simulink model "BenchmarkModel_Phasor_TestCase"  (R2020a)
settings: Solver=daessc  StartTime=0.0  StopTime=24*3600  RelTol=1e-2
undefined symbols (not defined in the file): A, a, Ac, B, Bc, C, Cc, Dc, Dd, find_system, Fnom, gcbh, I21_init_imag, I21_init_real, Ibase1, Ibase2, Iw1A_init_mag, Iw1A_init_pha, Iw1B_init_mag, Iw1B_init_pha, Iw1C_init_mag, Iw1C_init_pha, Iw2A_init_mag, Iw2A_init_pha, Iw2B_init_mag, Iw2B_init_pha, Iw2C_init_mag, Iw2C_init_pha, j, kr, ks, Nmax, Pnom, psi, sps_rtmsupport, V2G, Vnom1, Vnom2, w, Z1pu, Z2pu, Ztpu
libraries: powerlib x66, simulink x7, powerlib_meascontrol x7
(part 1 of 3)
settings Model: Creator=user  LastModifiedBy=anton
settings SolverCC: ZeroCrossControl=DisableAll

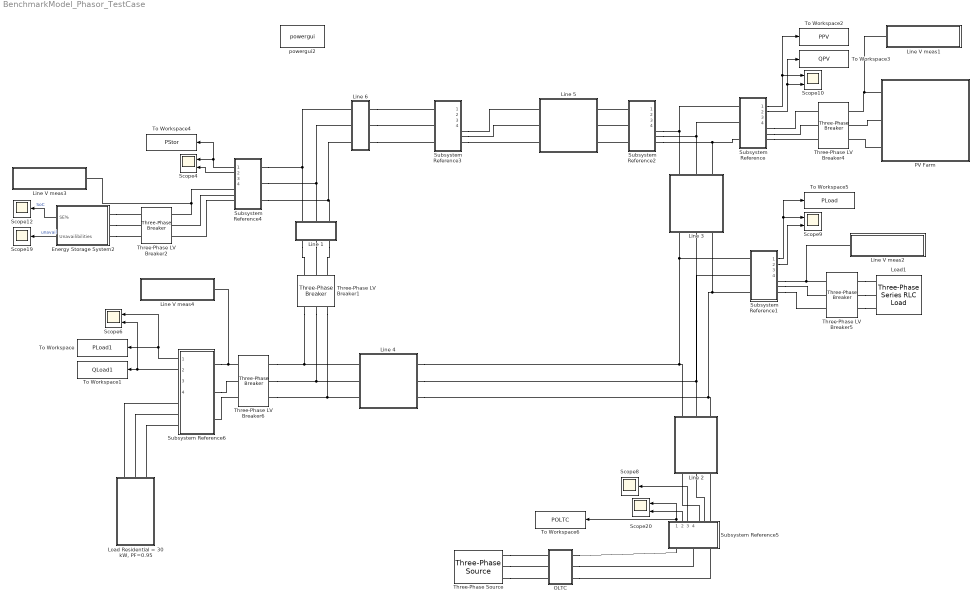
== system BenchmarkModel_Phasor_TestCase ==
  Energy Storage System2 : Subsystem  mask(Generic Energy Storage System){Pnom=15, kWh_Rated=75, Initial_kWh_pc=50, Efficiency=96, Pmax_Grid=27.5, Ki=100, MinMax=[ 10  90 ], ChargingPower=27.5}
      mask prompts: Pnom "Rated power in kW"; kWh_Rated "Rated capacity in kWh"; Initial_kWh_pc "Initial stored energy in % of rated capacity"; Efficiency "System efficiency in %"; Pmax_Grid "Maximum power allowed from the grid (kW)"; Ki "Regulator integral gain:"; MinMax "Range of operation [ min  max ] in % of Stored Energy"; ChargingPower "Maximum charging power (kW) during night time:"
      mask help:
      | Model a generic Energy Storage System (ESS) connected to grid through an inverter. The storage technology can be Battery, Flywheel, SuperCapacitor, ...
      |
      | Look Under Mask to see how the model is built.
      mask init:
      | Min=MinMax(1);
      | Max=MinMax(2);
      | Plimit=Pnom*1e3;
      mask DialogControl Container4 Prompt: Power
      mask DialogControl Container7 Prompt: Control
      mask Display: image(imread('Energy.jpg'))
  Line 1 : Subsystem  mask{Rline=0.497*3, Lline=0.086*3/(2*pi*50)}
      mask prompts: Rline "Resistance"; Lline "Reactance"
      mask DialogControl DescTextVar Prompt: Line block for LV grid
  Line 2 : Subsystem  mask{Rline=0.497*0.5, Lline=0.086*0.5/(2*pi*50)}
      mask prompts: Rline "Resistance"; Lline "Reactance"
      mask DialogControl DescTextVar Prompt: Line block for LV grid
  Line 3 : Subsystem  mask{Rline=0.497*2, Lline=0.086*2/(2*pi*50)}
      mask prompts: Rline "Resistance"; Lline "Reactance"
      mask DialogControl DescTextVar Prompt: Line block for LV grid
  Line 4 : Subsystem  mask{Rline=0.497*3, Lline=0.086*3/(2*pi*50)}
      mask prompts: Rline "Resistance"; Lline "Reactance"
      mask DialogControl DescTextVar Prompt: Line block for LV grid
  Line 5 : Subsystem  mask{Rline=0.497, Lline=0.086/(2*pi*50)}
      mask prompts: Rline "Resistance"; Lline "Reactance"
      mask DialogControl DescTextVar Prompt: Line block for LV grid
  Line 6 : Subsystem  mask{Rline=0.497, Lline=0.086/(2*pi*50)}
      mask prompts: Rline "Resistance"; Lline "Reactance"
      mask DialogControl DescTextVar Prompt: Line block for LV grid
  Line V meas1 : Subsystem
  Line V meas2 : Subsystem
  Line V meas3 : Subsystem
  Line V meas4 : Subsystem
  "Load Residential = 30 kW, PF=0.95" : Subsystem
      mask Display: image(imread('load.jpg'))
  Load1 : powerlib/Elements/Three-Phase Series RLC Load  LConnTagsString=A|B|C  Configuration=Y (grounded)  NominalVoltage=420  Vabc=[1e3 1e3 1e3]  Vabcp=[1e3 1e3 1e3]  NominalFrequency=50  UnbalancedPower=off  ActivePower=10e3  InductivePower=1e3  CapacitivePower=0  Pabc=[10e3 9e3 11e3]  QLabc=[100 90 110]  QCabc=[100 90 110]  Pabcp=[10e3 9e3 11e3]  QLabcp=[100 90 110]  QCabcp=[100 90 110]  Measurements=None  LoadType=constant Z
  OLTC : Subsystem
  PV Farm : Subsystem
      mask Display: image(imread('PV_Farm.jpg'))
  Scope{4,6,9..10,20} (5 alike) : Scope  NumInputPorts=2
  Scope12 : Scope
  Scope19 : Scope
  Scope8 : Scope
  Subsystem Reference{,1..6} (7 alike) : Subsystem  ReferencedSubsystem=Bus_phasor
  Three-Phase LV Breaker1 : powerlib/Elements/Three-Phase Breaker  InitialState=closed  SwitchA=on  SwitchB=on  SwitchC=on  SwitchTimes=[10*3600 10*3600+880]  External=off  BreakerResistance=0.001  SnubberResistance=1e5  SnubberCapacitance=inf  Measurements=None
  Three-Phase LV Breaker2 : powerlib/Elements/Three-Phase Breaker  InitialState=closed  SwitchA=on  SwitchB=on  SwitchC=on  SwitchTimes=1e9  External=off  BreakerResistance=0.001  SnubberResistance=1e5  SnubberCapacitance=inf  Measurements=None
  Three-Phase LV Breaker4 : powerlib/Elements/Three-Phase Breaker  InitialState=closed  SwitchA=on  SwitchB=on  SwitchC=on  SwitchTimes=25*3600  External=off  BreakerResistance=0.001  SnubberResistance=1e5  SnubberCapacitance=inf  Measurements=None
  Three-Phase LV Breaker5 : powerlib/Elements/Three-Phase Breaker  InitialState=closed  SwitchA=on  SwitchB=on  SwitchC=on  SwitchTimes=20*3600  External=off  BreakerResistance=0.001  SnubberResistance=1e5  SnubberCapacitance=inf  Measurements=None
  Three-Phase LV Breaker6 : powerlib/Elements/Three-Phase Breaker  InitialState=closed  SwitchA=on  SwitchB=on  SwitchC=on  SwitchTimes=1e10  External=off  BreakerResistance=0.001  SnubberResistance=1e5  SnubberCapacitance=inf  Measurements=None
  Three-Phase Source : powerlib/Electrical Sources/Three-Phase Source  InternalConnection=Yg  VoltagePhases=off  Voltage=20e3  PhaseAngle=0  Voltage_phases=[25e3 25e3 25e3]/sqrt(3)  PhaseAngles_phases=[0 -120 +120]  Frequency=50  NonIdealSource=on  SpecifyImpedance=off  Resistance=0.6145770  Inductance=0.00163022  ShortCircuitLevel=100e6  BaseVoltage=20e3  XRratio=7  BusType=swing  Pref=10e3  Qref=0  Prefabc=[10e3, 10e3, 10e3]  Qrefabc=[0, 0, 0]  Qmin=-inf  Qmax=inf
  To Workspace : ToWorkspace  VariableName=PLoad1  SaveFormat=Timeseries  SampleTime=-1
  To Workspace1 : ToWorkspace  VariableName=QLoad1  SaveFormat=Timeseries  SampleTime=-1
  To Workspace2 : ToWorkspace  VariableName=PPV  SaveFormat=Timeseries  SampleTime=-1
  To Workspace3 : ToWorkspace  VariableName=QPV  SaveFormat=Timeseries  SampleTime=-1
  To Workspace4 : ToWorkspace  VariableName=PStor  SaveFormat=Timeseries  SampleTime=-1
  To Workspace5 : ToWorkspace  VariableName=PLoad  SaveFormat=Timeseries  SampleTime=-1
  To Workspace6 : ToWorkspace  VariableName=POLTC  SaveFormat=Timeseries  SampleTime=-1
  powergui2 : powerlib/powergui  Priority=1  SimulationMode=Phasor  SampleTime=50e-6  frequency=50  Iterations=50  frequencyindice=50  Pbase=100e6  ErrMax=1e-4  UnitsV=kV  UnitsW=MW  buscounter=0  FunctionMessages=off  echomessages=off  EnableUseOfTLC=off  CurrentSourceSwitches=off  DisableSnubberDevices=off  DisableRonSwitches=off  DisableVfSwitches=off  DisplayEquations=off  AutomaticDiscreteSolvers=off  SolverType=Tustin/Backward Euler (TBE)  Interpol=off  ExternalGateDelay=off  methode=off  Ts=100  x0status=blocks  SPID=on  SwTol=0  HookPort=off  NonlinearTolerance=1e-4  nMaxIteration=100  ContinueOnMaxIteration=off  RestoreLinks=warning  ResistiveCurrentMeasurement=off  Frange=[0:2:500]  Ylog=off  Xlog=on  ShowGrid=off  save=off  variable=ZData  structure=0  ZoomFFT=off  StartTime=0.0  cycles=1  DisplayStyle=1  fundamental=60  FreqAxis=off  MaxFrequency=1000  frequencyindicesteady=1  RmsSteady=1  display=off
  wires:
  Subsystem Reference4/1 -> To Workspace4/1, Scope4/1
  Subsystem Reference4/2 -> Scope4/2
  Subsystem Reference1/2 -> Scope9/2
  Subsystem Reference1/1 -> To Workspace5/1, Scope9/1
  Subsystem Reference/1 -> To Workspace2/1, Scope10/1
  Subsystem Reference/2 -> To Workspace3/1, Scope10/2
  Energy Storage System2/1(SE%) -> Scope12/1  "SoC"
  Energy Storage System2/2(Unavailibilities) -> Scope19/1  "unavail"
  Subsystem Reference5/1 -> Scope20/1, To Workspace6/1
  Subsystem Reference5/2 -> Scope20/2
  Subsystem Reference6/1 -> Scope6/1, To Workspace/1
  Subsystem Reference6/2 -> Scope6/2, To Workspace1/1
  Subsystem Reference5/3 -> Scope8/1
  connections:
  Subsystem Reference2/RConn2 -- Subsystem Reference/LConn2 -- Line 3/LConn2
  Subsystem Reference1/LConn3 -- Line 4/LConn3 -- Line 2/LConn3 -- Line 3/RConn3
  OLTC/RConn2 -- Subsystem Reference5/LConn2
  OLTC/RConn3 -- Subsystem Reference5/LConn3
  Subsystem Reference3/RConn3 -- Line 5/RConn3
  Subsystem Reference3/RConn2 -- Line 5/RConn2
  Subsystem Reference3/RConn1 -- Line 5/RConn1
  Subsystem Reference2/LConn3 -- Line 5/LConn3
  Subsystem Reference2/LConn2 -- Line 5/LConn2
  Subsystem Reference2/LConn1 -- Line 5/LConn1
  Subsystem Reference4/LConn3 -- Line 6/LConn3 -- Line 1/LConn3
  Subsystem Reference4/LConn2 -- Line 1/LConn2 -- Line 6/LConn2
  Subsystem Reference4/LConn1 -- Line 1/LConn1 -- Line 6/LConn1
  Line 1/RConn2 -- Three-Phase LV Breaker1/RConn2
  Line 1/RConn1 -- Three-Phase LV Breaker1/RConn1
  Line 1/RConn3 -- Three-Phase LV Breaker1/RConn3
  Subsystem Reference2/RConn1 -- Subsystem Reference/LConn1 -- Line 3/LConn1
  Three-Phase LV Breaker1/LConn2 -- Three-Phase LV Breaker6/RConn2 -- Line 4/RConn2
  Three-Phase LV Breaker1/LConn1 -- Line 4/RConn1 -- Three-Phase LV Breaker6/RConn1
  Three-Phase LV Breaker1/LConn3 -- Line 4/RConn3 -- Three-Phase LV Breaker6/RConn3
  Energy Storage System2/LConn1 -- Three-Phase LV Breaker2/LConn1
  Energy Storage System2/LConn2 -- Three-Phase LV Breaker2/LConn2
  Energy Storage System2/LConn3 -- Three-Phase LV Breaker2/LConn3
  Subsystem Reference4/RConn1 -- Line V meas3/LConn1 -- Three-Phase LV Breaker2/RConn1
  Subsystem Reference4/RConn2 -- Three-Phase LV Breaker2/RConn2
  Subsystem Reference4/RConn3 -- Three-Phase LV Breaker2/RConn3
  PV Farm/RConn2 -- Three-Phase LV Breaker4/LConn2
  PV Farm/RConn3 -- Three-Phase LV Breaker4/LConn3
  Subsystem Reference/RConn1 -- Three-Phase LV Breaker4/RConn1
  Subsystem Reference/RConn2 -- Three-Phase LV Breaker4/RConn2
  Subsystem Reference/RConn3 -- Three-Phase LV Breaker4/RConn3
  Three-Phase LV Breaker5/LConn1 -- Load1/LConn1
  Three-Phase LV Breaker5/LConn2 -- Load1/LConn2
  Three-Phase LV Breaker5/LConn3 -- Load1/LConn3
  Subsystem Reference1/RConn1 -- Line V meas2/LConn1 -- Three-Phase LV Breaker5/RConn1
  Subsystem Reference1/RConn2 -- Three-Phase LV Breaker5/RConn2
  Subsystem Reference1/RConn3 -- Three-Phase LV Breaker5/RConn3
  "Load Residential = 30 kW, PF=0.95"/LConn1 -- Subsystem Reference6/RConn1
  "Load Residential = 30 kW, PF=0.95"/LConn2 -- Subsystem Reference6/RConn2
  "Load Residential = 30 kW, PF=0.95"/LConn3 -- Subsystem Reference6/RConn3
  Three-Phase Source/RConn1 -- OLTC/LConn1
  Three-Phase Source/RConn2 -- OLTC/LConn2
  Three-Phase Source/RConn3 -- OLTC/LConn3
  Subsystem Reference6/LConn1 -- Line V meas4/LConn1 -- Three-Phase LV Breaker6/LConn1
  Subsystem Reference6/LConn2 -- Three-Phase LV Breaker6/LConn2
  Subsystem Reference6/LConn3 -- Three-Phase LV Breaker6/LConn3
  PV Farm/RConn1 -- Line V meas1/LConn1 -- Three-Phase LV Breaker4/LConn1
  Subsystem Reference5/RConn3 -- Line 2/RConn3
  Subsystem Reference5/RConn2 -- Line 2/RConn2
  Subsystem Reference5/RConn1 -- Line 2/RConn1
  Line 2/LConn1 -- Subsystem Reference1/LConn1 -- Line 3/RConn1 -- Line 4/LConn1
  Subsystem Reference2/RConn3 -- Line 3/LConn3 -- Subsystem Reference/LConn3
  Line 4/LConn2 -- Subsystem Reference1/LConn2 -- Line 3/RConn2 -- Line 2/LConn2
  Line 6/RConn1 -- Subsystem Reference3/LConn1
  Line 6/RConn2 -- Subsystem Reference3/LConn2
  Line 6/RConn3 -- Subsystem Reference3/LConn3
  OLTC/RConn1 -- Subsystem Reference5/LConn1

== system BenchmarkModel_Phasor_TestCase/Energy Storage System2 ==
  Compute number of unavailibilities : Subsystem
  ESS Control : Subsystem
  Gain : Gain  Gain=-1
  Inverter (Phasor) : Subsystem
  On=1 : Step  Time=0.01*24*60*60  Before=1  SampleTime=0
  Saturation : Saturate  UpperLimit=Pnom*1e3  LowerLimit=-Pnom*1e3
  Scope : Scope
  Stored Energy Calculation (%) : Subsystem
  A : PMIOPort  Tag=PMCPort  Side=Left
  B : PMIOPort  Tag=PMCPort  Port=2  Side=Left
  C : PMIOPort  Tag=PMCPort  Port=3  Side=Left
  SE% : Outport
  Unavailibilities : Outport  Port=2
  wires:
  Saturation/1 -> Gain/1, Inverter (Phasor)/1(Power), Stored Energy Calculation (%)/1(Pin), Compute number of unavailibilities/2(Sat Out)
  ESS Control/1(P) -> Saturation/1, Compute number of unavailibilities/1(Sat In)
  [Vabc_B1] -> ESS Control/1(Vabc)
  [Iabc_B1] -> ESS Control/2(Iabc)
  On=1/1 -> ESS Control/3(On)
  ESS Control/2(LessThan Min) -> Compute number of unavailibilities/3(LessThanMin)
  Compute number of unavailibilities/1(Unavailibilities) -> Unavailibilities/1
  Stored Energy Calculation (%)/1(SE%) -> SE%/1, ESS Control/4(SE%)
  Gain/1 -> Scope/1
  connections:
  Inverter (Phasor)/RConn1 -- A/RConn1
  Inverter (Phasor)/RConn2 -- B/RConn1
  Inverter (Phasor)/RConn3 -- C/RConn1

== system BenchmarkModel_Phasor_TestCase/Line 1 ==
  Series RLC BranchA : powerlib/Elements/Series RLC Branch  LConnTagsString=__new0  RConnTagsString=__new0  BranchType=RL  Resistance=Rline  Inductance=Lline  SetiL0=off  InitialCurrent=0  Capacitance=1e-6  Setx0=off  InitialVoltage=0  Measurements=None
  Series RLC BranchB : powerlib/Elements/Series RLC Branch  LConnTagsString=__new0  RConnTagsString=__new0  BranchType=RL  Resistance=Rline  Inductance=Lline  SetiL0=off  InitialCurrent=0  Capacitance=1e-6  Setx0=off  InitialVoltage=0  Measurements=None
  Series RLC BranchC : powerlib/Elements/Series RLC Branch  LConnTagsString=__new0  RConnTagsString=__new0  BranchType=RL  Resistance=Rline  Inductance=Lline  SetiL0=off  InitialCurrent=0  Capacitance=1e-6  Setx0=off  InitialVoltage=0  Measurements=None
  a : PMIOPort  Side=Left
  A : PMIOPort  Port=2  Side=Right
  b : PMIOPort  Port=3  Side=Left
  B : PMIOPort  Port=4  Side=Right
  c : PMIOPort  Port=5  Side=Left
  C : PMIOPort  Port=6  Side=Right
  connections:
  Series RLC BranchB/RConn1 -- B/RConn1
  Series RLC BranchC/RConn1 -- C/RConn1
  Series RLC BranchB/LConn1 -- b/RConn1
  Series RLC BranchA/RConn1 -- A/RConn1
  Series RLC BranchA/LConn1 -- a/RConn1
  Series RLC BranchC/LConn1 -- c/RConn1

== system BenchmarkModel_Phasor_TestCase/Line 2 ==
  Series RLC BranchA : powerlib/Elements/Series RLC Branch  LConnTagsString=__new0  RConnTagsString=__new0  BranchType=RL  Resistance=Rline  Inductance=Lline  SetiL0=off  InitialCurrent=0  Capacitance=1e-6  Setx0=off  InitialVoltage=0  Measurements=None
  Series RLC BranchB : powerlib/Elements/Series RLC Branch  LConnTagsString=__new0  RConnTagsString=__new0  BranchType=RL  Resistance=Rline  Inductance=Lline  SetiL0=off  InitialCurrent=0  Capacitance=1e-6  Setx0=off  InitialVoltage=0  Measurements=None
  Series RLC BranchC : powerlib/Elements/Series RLC Branch  LConnTagsString=__new0  RConnTagsString=__new0  BranchType=RL  Resistance=Rline  Inductance=Lline  SetiL0=off  InitialCurrent=0  Capacitance=1e-6  Setx0=off  InitialVoltage=0  Measurements=None
  a : PMIOPort  Side=Left
  A : PMIOPort  Port=2  Side=Right
  b : PMIOPort  Port=3  Side=Left
  B : PMIOPort  Port=4  Side=Right
  c : PMIOPort  Port=5  Side=Left
  C : PMIOPort  Port=6  Side=Right
  connections:
  Series RLC BranchC/LConn1 -- c/RConn1
  Series RLC BranchA/LConn1 -- a/RConn1
  Series RLC BranchA/RConn1 -- A/RConn1
  Series RLC BranchB/LConn1 -- b/RConn1
  Series RLC BranchC/RConn1 -- C/RConn1
  Series RLC BranchB/RConn1 -- B/RConn1

== system BenchmarkModel_Phasor_TestCase/Line 3 ==
  Series RLC BranchA : powerlib/Elements/Series RLC Branch  LConnTagsString=__new0  RConnTagsString=__new0  BranchType=RL  Resistance=Rline  Inductance=Lline  SetiL0=off  InitialCurrent=0  Capacitance=1e-6  Setx0=off  InitialVoltage=0  Measurements=None
  Series RLC BranchB : powerlib/Elements/Series RLC Branch  LConnTagsString=__new0  RConnTagsString=__new0  BranchType=RL  Resistance=Rline  Inductance=Lline  SetiL0=off  InitialCurrent=0  Capacitance=1e-6  Setx0=off  InitialVoltage=0  Measurements=None
  Series RLC BranchC : powerlib/Elements/Series RLC Branch  LConnTagsString=__new0  RConnTagsString=__new0  BranchType=RL  Resistance=Rline  Inductance=Lline  SetiL0=off  InitialCurrent=0  Capacitance=1e-6  Setx0=off  InitialVoltage=0  Measurements=None
  a : PMIOPort  Side=Left
  A : PMIOPort  Port=2  Side=Right
  b : PMIOPort  Port=3  Side=Left
  B : PMIOPort  Port=4  Side=Right
  c : PMIOPort  Port=5  Side=Left
  C : PMIOPort  Port=6  Side=Right
  connections:
  Series RLC BranchB/RConn1 -- B/RConn1
  Series RLC BranchC/RConn1 -- C/RConn1
  Series RLC BranchB/LConn1 -- b/RConn1
  Series RLC BranchA/RConn1 -- A/RConn1
  Series RLC BranchA/LConn1 -- a/RConn1
  Series RLC BranchC/LConn1 -- c/RConn1

== system BenchmarkModel_Phasor_TestCase/Line 4 ==
  Series RLC BranchA : powerlib/Elements/Series RLC Branch  LConnTagsString=__new0  RConnTagsString=__new0  BranchType=RL  Resistance=Rline  Inductance=Lline  SetiL0=off  InitialCurrent=0  Capacitance=1e-6  Setx0=off  InitialVoltage=0  Measurements=None
  Series RLC BranchB : powerlib/Elements/Series RLC Branch  LConnTagsString=__new0  RConnTagsString=__new0  BranchType=RL  Resistance=Rline  Inductance=Lline  SetiL0=off  InitialCurrent=0  Capacitance=1e-6  Setx0=off  InitialVoltage=0  Measurements=None
  Series RLC BranchC : powerlib/Elements/Series RLC Branch  LConnTagsString=__new0  RConnTagsString=__new0  BranchType=RL  Resistance=Rline  Inductance=Lline  SetiL0=off  InitialCurrent=0  Capacitance=1e-6  Setx0=off  InitialVoltage=0  Measurements=None
  a : PMIOPort  Side=Left
  A : PMIOPort  Port=2  Side=Right
  b : PMIOPort  Port=3  Side=Left
  B : PMIOPort  Port=4  Side=Right
  c : PMIOPort  Port=5  Side=Left
  C : PMIOPort  Port=6  Side=Right
  connections:
  Series RLC BranchB/RConn1 -- B/RConn1
  Series RLC BranchC/RConn1 -- C/RConn1
  Series RLC BranchB/LConn1 -- b/RConn1
  Series RLC BranchA/RConn1 -- A/RConn1
  Series RLC BranchA/LConn1 -- a/RConn1
  Series RLC BranchC/LConn1 -- c/RConn1

== system BenchmarkModel_Phasor_TestCase/Line 5 ==
  Series RLC BranchA : powerlib/Elements/Series RLC Branch  LConnTagsString=__new0  RConnTagsString=__new0  BranchType=RL  Resistance=Rline  Inductance=Lline  SetiL0=off  InitialCurrent=0  Capacitance=1e-6  Setx0=off  InitialVoltage=0  Measurements=None
  Series RLC BranchB : powerlib/Elements/Series RLC Branch  LConnTagsString=__new0  RConnTagsString=__new0  BranchType=RL  Resistance=Rline  Inductance=Lline  SetiL0=off  InitialCurrent=0  Capacitance=1e-6  Setx0=off  InitialVoltage=0  Measurements=None
  Series RLC BranchC : powerlib/Elements/Series RLC Branch  LConnTagsString=__new0  RConnTagsString=__new0  BranchType=RL  Resistance=Rline  Inductance=Lline  SetiL0=off  InitialCurrent=0  Capacitance=1e-6  Setx0=off  InitialVoltage=0  Measurements=None
  a : PMIOPort  Side=Left
  A : PMIOPort  Port=2  Side=Right
  b : PMIOPort  Port=3  Side=Left
  B : PMIOPort  Port=4  Side=Right
  c : PMIOPort  Port=5  Side=Left
  C : PMIOPort  Port=6  Side=Right
  connections:
  Series RLC BranchB/RConn1 -- B/RConn1
  Series RLC BranchC/RConn1 -- C/RConn1
  Series RLC BranchB/LConn1 -- b/RConn1
  Series RLC BranchA/RConn1 -- A/RConn1
  Series RLC BranchA/LConn1 -- a/RConn1
  Series RLC BranchC/LConn1 -- c/RConn1

== system BenchmarkModel_Phasor_TestCase/Line 6 ==
  Series RLC BranchA : powerlib/Elements/Series RLC Branch  LConnTagsString=__new0  RConnTagsString=__new0  BranchType=RL  Resistance=Rline  Inductance=Lline  SetiL0=off  InitialCurrent=0  Capacitance=1e-6  Setx0=off  InitialVoltage=0  Measurements=None
  Series RLC BranchB : powerlib/Elements/Series RLC Branch  LConnTagsString=__new0  RConnTagsString=__new0  BranchType=RL  Resistance=Rline  Inductance=Lline  SetiL0=off  InitialCurrent=0  Capacitance=1e-6  Setx0=off  InitialVoltage=0  Measurements=None
  Series RLC BranchC : powerlib/Elements/Series RLC Branch  LConnTagsString=__new0  RConnTagsString=__new0  BranchType=RL  Resistance=Rline  Inductance=Lline  SetiL0=off  InitialCurrent=0  Capacitance=1e-6  Setx0=off  InitialVoltage=0  Measurements=None
  a : PMIOPort  Side=Left
  A : PMIOPort  Port=2  Side=Right
  b : PMIOPort  Port=3  Side=Left
  B : PMIOPort  Port=4  Side=Right
  c : PMIOPort  Port=5  Side=Left
  C : PMIOPort  Port=6  Side=Right
  connections:
  Series RLC BranchB/RConn1 -- B/RConn1
  Series RLC BranchC/RConn1 -- C/RConn1
  Series RLC BranchB/LConn1 -- b/RConn1
  Series RLC BranchA/RConn1 -- A/RConn1
  Series RLC BranchA/LConn1 -- a/RConn1
  Series RLC BranchC/LConn1 -- c/RConn1

== system BenchmarkModel_Phasor_TestCase/Line V meas1 ==
  To Workspace4 : ToWorkspace  VariableName=VmagPV  SaveFormat=Timeseries  SampleTime=-1
  Va (V)2 : Scope
  Va2 : powerlib/Measurements/Voltage Measurement  Tag=PoWeRsYsTeMmEaSuReMeNt  PhasorSimulation=on  OutputType=Magnitude  PSBequivalent=0
  output Ground3 : powerlib/Elements/Ground  LConnTagsString=a
  + : PMIOPort  Side=Left
  wires:
  Va2/1 -> To Workspace4/1, Va (V)2/1  "ASM terminal voltage"
  connections:
  output Ground3/LConn1 -- Va2/LConn2
  Va2/LConn1 -- +/RConn1

== system BenchmarkModel_Phasor_TestCase/Line V meas2 ==
  To Workspace4 : ToWorkspace  VariableName=VmagLoad  SaveFormat=Timeseries  SampleTime=-1
  Va (V)2 : Scope
  Va2 : powerlib/Measurements/Voltage Measurement  Tag=PoWeRsYsTeMmEaSuReMeNt  PhasorSimulation=on  OutputType=Magnitude  PSBequivalent=0
  output Ground3 : powerlib/Elements/Ground  LConnTagsString=a
  + : PMIOPort  Side=Left
  wires:
  Va2/1 -> To Workspace4/1, Va (V)2/1  "ASM terminal voltage"
  connections:
  output Ground3/LConn1 -- Va2/LConn2
  Va2/LConn1 -- +/RConn1

== system BenchmarkModel_Phasor_TestCase/Line V meas3 ==
  To Workspace4 : ToWorkspace  VariableName=VmagStor  SaveFormat=Timeseries  SampleTime=-1
  Va (V)2 : Scope
  Va2 : powerlib/Measurements/Voltage Measurement  Tag=PoWeRsYsTeMmEaSuReMeNt  PhasorSimulation=on  OutputType=Magnitude  PSBequivalent=0
  output Ground3 : powerlib/Elements/Ground  LConnTagsString=a
  + : PMIOPort  Side=Left
  wires:
  Va2/1 -> To Workspace4/1, Va (V)2/1  "ASM terminal voltage"
  connections:
  output Ground3/LConn1 -- Va2/LConn2
  Va2/LConn1 -- +/RConn1

== system BenchmarkModel_Phasor_TestCase/Line V meas4 ==
  To Workspace4 : ToWorkspace  VariableName=VmagLoad1  SaveFormat=Timeseries  SampleTime=-1
  Va (V)2 : Scope
  Va2 : powerlib/Measurements/Voltage Measurement  Tag=PoWeRsYsTeMmEaSuReMeNt  PhasorSimulation=on  OutputType=Magnitude  PSBequivalent=0
  output Ground3 : powerlib/Elements/Ground  LConnTagsString=a
  + : PMIOPort  Side=Left
  wires:
  Va2/1 -> To Workspace4/1, Va (V)2/1  "ASM terminal voltage"
  connections:
  output Ground3/LConn1 -- Va2/LConn2
  Va2/LConn1 -- +/RConn1

== system BenchmarkModel_Phasor_TestCase/Load Residential = 30 kW, PF=0.95 ==
  Residential Load1 : Subsystem  mask{nomPower=30, PF=0.95, timestep=15}
      mask prompts: nomPower "Nominal Power (kW)"; PF "Power factor"; timestep "Timestep (minutes)"
      mask DialogControl DescGroupVar Prompt: Load profile
      mask DialogControl DescTextVar Prompt: The load profile allows you to fix a nominal power and and a power factor. It is also needed to specify the timestep used for the consumption datas. Finally, a vector expresses the consumption profile. It has to be expressed in per unit. It is imperative that the length of the vector fits with the timestep used.
      mask Display: image(imread('Residential.jpg'))
  A : PMIOPort  Side=Left
  B : PMIOPort  Port=2  Side=Left
  C : PMIOPort  Port=3  Side=Left
  connections:
  Residential Load1/LConn1 -- A/RConn1
  Residential Load1/LConn2 -- B/RConn1
  Residential Load1/LConn3 -- C/RConn1

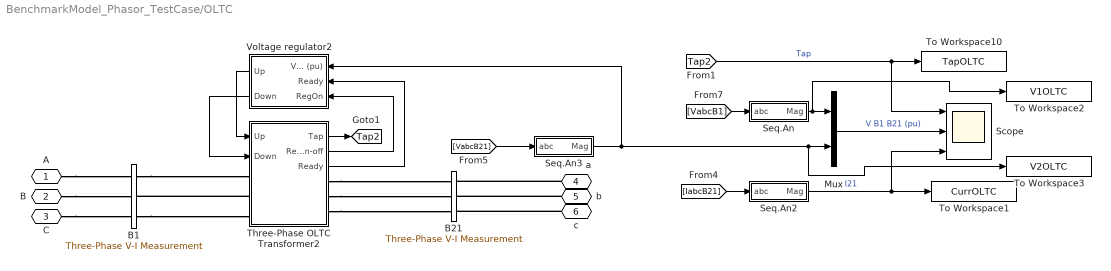
== system BenchmarkModel_Phasor_TestCase/OLTC ==
  B1 : powerlib/Measurements/Three-Phase V-I Measurement  VoltageMeasurement=phase-to-ground  SetLabelV=on  LabelV=VabcB1  Vpu=on  VpuLL=off  CurrentMeasurement=yes  SetLabelI=on  LabelI=IabcB1  Ipu=on  Pbase=630e3  Vbase=20000  OutputType=Complex  PhasorSimulation=on  PSBequivalent=0
  B21 : powerlib/Measurements/Three-Phase V-I Measurement  VoltageMeasurement=phase-to-ground  SetLabelV=on  LabelV=VabcB21  Vpu=on  VpuLL=off  CurrentMeasurement=yes  SetLabelI=on  LabelI=IabcB21  Ipu=on  Pbase=630e3  Vbase=420  OutputType=Complex  PhasorSimulation=on  PSBequivalent=0
  Mux : Mux  Inputs=2
  Scope : Scope  NumInputPorts=3
  Seq.An : Subsystem
  Seq.An2 : Subsystem
  Seq.An3 : Subsystem
  Three-Phase OLTC Transformer2 : Subsystem  AncestorBlock=|  DialogController=POWERSYS.PowerSysDialog  LoadFcn=sps_rtmsupport('LoadFcn',gcbh); %find_system(gcs,'FollowLinks', 'on', 'LookUnderMasks', 'all');  StartFcn=sps_rtmsupport('StartFcn',gcbh);  StopFcn=sps_rtmsupport('StopFcn',gcbh);  mask(Three-Phase OLTC Regulating Transformer (Phasor Type)){Winding1Connection=Delta (D11), Winding2Connection=Y, PnomFnom=[250e3  50], Winding1=[20000  0.003 0.09 ], Winding2=[420   0.003 0.09 ], Iw2_init=[0.15 -50], RmXm=[300 300], TapOnWinding=Winding 1, WindingTap=[ 0.003 0.09], dU=0.01875/5, TapMinMax=[ -8  +8], InitialTap=-4, TapSelectionTime=10, ExternalControl=on, RegulatorOn=on, Regulator=[1.04   0.0375 1]}
      | spsThreePhaseOLTCRegulatingTransformerPhasorTypeLib/Three-Phase OLTC
      | Regulating Transformer
      | (Phasor Type)
      mask prompts: Winding1Connection "Winding 1 connection (ABC terminals):"; Winding2Connection "Winding 2 connection (abc terminals):"; PnomFnom "Nominal power and frequency [Pn(VA), fn(Hz)]"; Winding1 "Winding 1 parameters [V1 Ph-Ph(Vrms), R1(pu),  X1(pu)]"; Winding2 "Winding 2 parameters [V2 Ph-Ph(Vrms),  R2(pu),  X2(pu)]"; Iw2_init "Initial pos. seq. output currents of winding 2 [Mag(pu),  Phase(deg)]"; RmXm "Magnetization branch [Rm(pu)  Xm(pu)]"; TapOnWinding "OLTC on:"; WindingTap "Tapped regulation winding [Rt(pu),  Xt(pu)]"; dU "Voltage step per tap (pu)"; TapMinMax "Minimum and maximum tap positions [Min, Max]"; InitialTap "Initial tap position"; TapSelectionTime "Tap selection time (s)"; ExternalControl "External control of OLTC"; RegulatorOn "Voltage regulator"; Regulator "Regulator parameters [ Vref(pu) DeadBand(pu)  Delay(s)]"
      mask help: Implement phasor model of three-phase OLTC regulating transformer. It consists of two fixed windings and a third tapped winding (regulation winding) connected in series with either winding 1 or winding 2. Voltage ratio and transformer impedance vary with tap position. A +30 degrees or -30 degrees phase shift is introduced when winding 1 or winding 2 are connected in Delta.
      mask init:
      | [a,Z1pu,Z2pu,Ztpu,psi,ks,kr,RegulatorVref, RegulatorDeadBand,RegulatorDelay,Iw2A_init_mag,Iw2B_init_mag,Iw2C_init_mag, Iw2A_init_pha,Iw2B_init_pha,Iw2C_init_pha,N2_N1,Iw1A_init_mag,Iw1B_init_mag,Iw1C_init_mag,Iw1A_init_pha,Iw1B_init_pha,Iw1C_init_pha,I21_init_real,I21_init_imag,Nmax,w,Vnom1,Vnom2,Ibase1,Ibase2,Pnom,Fnom ] = powericon('OLTCRegulatingTansformerInit',InitialTap, TapMinMax,PnomFnom,Winding1,Winding1Connection,Winding2,Winding2Connection,Regulator,Iw2_init,TapOnWinding,dU,WindingTap);
      | OLTCtransformerCback(gcbh,2);
      | power_initmask();
      settings: CopyFcn=sps_rtmsupport('CopyFcn',gcbh);  DeleteFcn=sps_rtmsupport('DeleteFcn',gcbh);  UndoDeleteFcn=sps_rtmsupport('UndoDeleteFcn',gcbh);  ModelCloseFcn=sps_rtmsupport('ModelCloseFcn',gcbh);  PreSaveFcn=sps_rtmsupport('PreSaveFcn',gcbh);  PostSaveFcn=sps_rtmsupport('PostSaveFcn',gcbh);  NameChangeFcn=sps_rtmsupport('NameChangeFcn',gcbh);  PreCopyFcn=sps_rtmsupport('PreCopyFcn',gcbh);  OpenFcn=sps_rtmsupport('OpenFcn',gcbh, [1 2 8 14 15]);  CloseFcn=sps_rtmsupport('CloseFcn',gcbh);  PreDeleteFcn=sps_rtmsupport('PreDeleteFcn',gcbh);
      mask Help: helpview(psbhelp)
      mask TypeOptions Winding1Connection: Y | Yg | Delta (D1) | Delta (D11)
      mask TypeOptions Winding2Connection: Y | Yg | Delta (D1) | Delta (D11)
      mask TypeOptions TapOnWinding: Winding 1 | Winding 2
      mask Callback ExternalControl: %OLTCtransformerCback(gcbh,2);
      mask TypeOptions RegulatorOn: off | on
      mask Callback RegulatorOn: OLTCtransformerCback(gcbh,3);
      mask DialogControl Transformerparameters Prompt: Transformer
      mask DialogControl OLTCandVoltageRegulatorparameters Prompt: OLTC and Voltage Regulator
      mask Display: disp('')
  To Workspace1 : ToWorkspace  VariableName=CurrOLTC  SaveFormat=Timeseries  SampleTime=-1
  To Workspace10 : ToWorkspace  VariableName=TapOLTC  SaveFormat=Timeseries  SampleTime=-1
  To Workspace2 : ToWorkspace  VariableName=V1OLTC  SaveFormat=Timeseries  SampleTime=-1
  To Workspace3 : ToWorkspace  VariableName=V2OLTC  SaveFormat=Timeseries  SampleTime=-1
  Voltage regulator2 : Subsystem  mask{Vref=1.0, DeadBand=0.01875/5, TimeDelay=3}
      mask prompts: Vref "Vref (pu)"; DeadBand "Deadband (pu)"; TimeDelay "Time delay (s)"
  A : PMIOPort  Side=Left
  B : PMIOPort  Port=2  Side=Left
  C : PMIOPort  Port=3  Side=Left
  a : PMIOPort  Port=4  Side=Right
  b : PMIOPort  Port=5  Side=Right
  c : PMIOPort  Port=6  Side=Right
  tag scope: Tap2=global
  wires:
  [VabcB21] -> Seq.An3/1(abc)
  Seq.An3/1(Mag) -> Voltage regulator2/1(Vmes (pu)), To Workspace3/1, Mux/2
  Three-Phase OLTC Transformer2/1(Tap) -> [Tap2]
  Mux/1 -> Scope/2  "V B1 B21 (pu)"
  Three-Phase OLTC Transformer2/2(Reg on-off) -> Voltage regulator2/3(RegOn)
  [Tap2] -> Scope/1, To Workspace10/1  "Tap"
  [VabcB1] -> Seq.An/1(abc)
  [IabcB21] -> Seq.An2/1(abc)
  Three-Phase OLTC Transformer2/3(Ready) -> Voltage regulator2/2(Ready)
  Seq.An/1(Mag) -> To Workspace2/1, Mux/1
  Seq.An2/1(Mag) -> Scope/3, To Workspace1/1  "I21"
  Voltage regulator2/1("Up ") -> Three-Phase OLTC Transformer2/1(Up)
  Voltage regulator2/2("Down ") -> Three-Phase OLTC Transformer2/2(Down)
  connections:
  Three-Phase OLTC Transformer2/RConn2 -- B21/LConn2
  Three-Phase OLTC Transformer2/RConn1 -- B21/LConn1
  Three-Phase OLTC Transformer2/RConn3 -- B21/LConn3
  B1/RConn3 -- Three-Phase OLTC Transformer2/LConn3
  c/RConn1 -- B21/RConn3
  Three-Phase OLTC Transformer2/LConn2 -- B1/RConn2
  C/RConn1 -- B1/LConn3
  B1/RConn1 -- Three-Phase OLTC Transformer2/LConn1
  B/RConn1 -- B1/LConn2
  b/RConn1 -- B21/RConn2
  A/RConn1 -- B1/LConn1
  a/RConn1 -- B21/RConn1

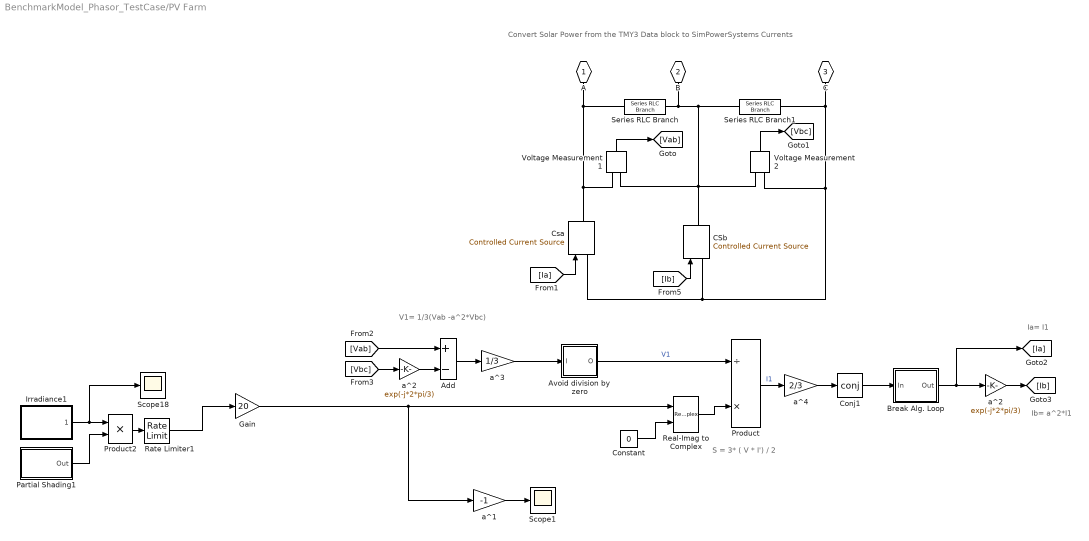
== system BenchmarkModel_Phasor_TestCase/PV Farm ==
  note: Ib= a^2*I1
  note: Ia= I1
  note: S = 3* ( V * I') / 2
  note: V1= 1/3(Vab -a^2*Vbc)
  note: Convert Solar Power from the TMY3 Data block to SimPowerSystems Currents
  Add : Sum  Inputs=+-
  Avoid division by zero : Subsystem
  "Break Alg. Loop " : Subsystem
  CSb : powerlib/Electrical Sources/Controlled Current Source  Initialize=off  Source_Type=AC  Amplitude=0  Phase=0  Frequency=0  Measurements=None
  Conj1 : Math  Operator=conj  SignedPower=on  SaturateOnIntegerOverflow=on
  Constant : Constant  Value=0
  Csa : powerlib/Electrical Sources/Controlled Current Source  Initialize=off  Source_Type=AC  Amplitude=0  Phase=0  Frequency=0  Measurements=None
  Gain : Gain  Gain=20
  Irradiance1 : Subsystem
      mask init:
      | load power_V2G
      mask Display: plot(V2G.IRRADIANCE.time,V2G.IRRADIANCE.SUN)
  Partial Shading1 : Subsystem  mask(Signal Disturbance){Hour=12, Minute=0, Second=0, Duration=5*60, Factor=0.7}
      mask prompts: Duration "Duration (s):"
      mask help: Within the specified time range defined by Start and Duration parameters, output is set to 'Factor'. Outside the specified time range output is kept at 1.0.
      mask init:
      | T2=(Hour-1)*60*60;    % Hour in seconds
      | T3=(Minute-1)*60;  % Minute in seconds
      | Ton=T2+T3+(Second-1);    % Beginning of fault (s)
      | Toff=Ton+Duration; % End of fault (s)
      mask TypeOptions Hour: 0 |      1 |      2 |      3 |      4 |      5 |      6 |      7 |      8 |      9 |     10 |     11 |     12 |     13 |     14 |     15 |     16 |     17 |     18 |     19 |     20 |     21 |     22 |     23
      mask TypeOptions Minute: 0 |      1 |      2 |      3 |      4 |      5 |      6 |      7 |      8 |      9 |     10 |     11 |     12 |     13 |     14 |     15 |     16 |     17 |     18 |     19 |     20 |     21 |     22 |     23 |     24 |     25 |     26 |     27 |     28 |     29 |     30 |     31 |     32 |     33 |     34 |     35 |     36 |     37 |     38 |     39 |     40 |     41 |     42 |     43 |     44 |     45 |     46 |     47 |     48 |     49 |     50 |     51 |     52 |     53 |     54 |     55 |     56 |     57 |     58 |     59
      mask TypeOptions Second: 0 |      1 |      2 |      3 |      4 |      5 |      6 |      7 |      8 |      9 |     10 |     11 |     12 |     13 |     14 |     15 |     16 |     17 |     18 |     19 |     20 |     21 |     22 |     23 |     24 |     25 |     26 |     27 |     28 |     29 |     30 |     31 |     32 |     33 |     34 |     35 |     36 |     37 |     38 |     39 |     40 |     41 |     42 |     43 |     44 |     45 |     46 |     47 |     48 |     49 |     50 |     51 |     52 |     53 |     54 |     55 |     56 |     57 |     58 |     59
      mask DialogControl Control2 Prompt: Start:
  Product : Product  Inputs=/*  InputSameDT=on  SaturateOnIntegerOverflow=on  OutDataTypeStr=Inherit: Same as first input
  Product2 : Product
  Rate Limiter1 : RateLimiter  RisingSlewLimit=1e4  FallingSlewLimit=-1e4  SampleTimeMode=inherited
  Real-Imag to Complex : RealImagToComplex
  Scope1 : Scope
  Scope18 : Scope
  Series RLC Branch : powerlib/Elements/Series RLC Branch  LConnTagsString=__new0  RConnTagsString=__new0  BranchType=R  Resistance=1e6  Inductance=1e-3  SetiL0=off  InitialCurrent=0  Capacitance=1e-6  Setx0=off  InitialVoltage=0  Measurements=None
  Series RLC Branch1 : powerlib/Elements/Series RLC Branch  LConnTagsString=__new0  RConnTagsString=__new0  BranchType=R  Resistance=1e6  Inductance=1e-3  SetiL0=off  InitialCurrent=0  Capacitance=1e-6  Setx0=off  InitialVoltage=0  Measurements=None
  Voltage Measurement1 : powerlib/Measurements/Voltage Measurement  PhasorSimulation=on  OutputType=Complex  PSBequivalent=0
  Voltage Measurement2 : powerlib/Measurements/Voltage Measurement  PhasorSimulation=on  OutputType=Complex  PSBequivalent=0
  a^1 : Gain  Gain=-1  SaturateOnIntegerOverflow=on  OutDataTypeStr=Inherit: Same as input  ParamDataTypeStr=Inherit: Same as input
  a^2 : Gain  Gain=exp(-j*2*pi/3)  SaturateOnIntegerOverflow=on  OutDataTypeStr=Inherit: Same as input  ParamDataTypeStr=Inherit: Same as input
  "a^2 " : Gain  Gain=exp(-j*2*pi/3)  SaturateOnIntegerOverflow=on  OutDataTypeStr=Inherit: Same as input  ParamDataTypeStr=Inherit: Same as input
  a^3 : Gain  Gain=1/3  SaturateOnIntegerOverflow=on  OutDataTypeStr=Inherit: Same as input  ParamDataTypeStr=Inherit: Same as input
  a^4 : Gain  Gain=2/3  SaturateOnIntegerOverflow=on  OutDataTypeStr=Inherit: Same as input  ParamDataTypeStr=Inherit: Same as input
  A : PMIOPort  Tag=PMCPort  Side=Right
  B : PMIOPort  Tag=PMCPort  Port=2  Side=Right
  C : PMIOPort  Tag=PMCPort  Port=3  Side=Right
  wires:
  [Ib] -> CSb/1
  "Break Alg. Loop "/1(Out) -> a^2/1, [Ia]
  a^4/1 -> Conj1/1
  "a^2 "/1 -> Add/2
  [Vbc] -> "a^2 "/1
  [Vab] -> Add/1
  Add/1 -> a^3/1
  a^3/1 -> Avoid division by zero/1(I)
  Conj1/1 -> "Break Alg. Loop "/1(In)
  Avoid division by zero/1(O) -> Product/1  "V1"
  a^2/1 -> [Ib]
  [Ia] -> Csa/1
  Product/1 -> a^4/1  "I1"
  Real-Imag to Complex/1 -> Product/2
  Voltage Measurement2/1 -> [Vbc]
  Voltage Measurement1/1 -> [Vab]
  Constant/1 -> Real-Imag to Complex/2
  Irradiance1/1(" ") -> Scope18/1, Product2/1
  Product2/1 -> Rate Limiter1/1
  Rate Limiter1/1 -> Gain/1
  Partial Shading1/1(Out) -> Product2/2
  Gain/1 -> a^1/1, Real-Imag to Complex/1
  a^1/1 -> Scope1/1
  connections:
  CSb/RConn1 -- Voltage Measurement1/LConn2 -- Voltage Measurement2/LConn1 -- Series RLC Branch/RConn1 -- B/RConn1 -- Series RLC Branch1/LConn1
  Voltage Measurement2/LConn2 -- Csa/LConn1 -- CSb/LConn1 -- C/RConn1 -- Series RLC Branch1/RConn1
  A/RConn1 -- Series RLC Branch/LConn1 -- Voltage Measurement1/LConn1 -- Csa/RConn1

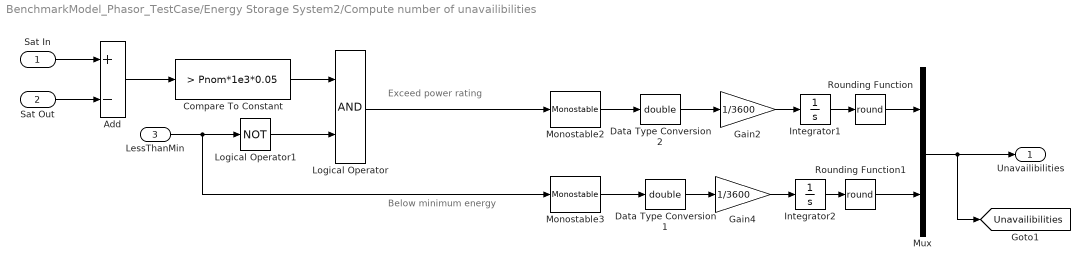
== system BenchmarkModel_Phasor_TestCase/Energy Storage System2/Compute number of unavailibilities ==
  note: Exceed power rating
  note: Below minimum energy
  Sat In : Inport
  Sat Out : Inport  Port=2
  LessThanMin : Inport  Port=3
  Add : Sum  Inputs=+-
  Compare To Constant : simulink/Logic and Bit Operations/Compare To Constant  relop=>  const=Pnom*1e3*0.05  OutDataTypeStr=uint8
  Data Type Conversion1 : DataTypeConversion  OutDataTypeStr=double
  Data Type Conversion2 : DataTypeConversion  OutDataTypeStr=double
  Gain2 : Gain  Gain=1/3600
  Gain4 : Gain  Gain=1/3600
  Integrator1 : Integrator
  Integrator2 : Integrator
  Logical Operator : Logic  AllPortsSameDT=off  OutDataTypeStr=boolean
  Logical Operator1 : Logic  Operator=NOT  AllPortsSameDT=off  OutDataTypeStr=boolean
  Monostable2 : powerlib_meascontrol/Logic/Monostable  EdgeDetect=Rising  PulseDuration=3600  ic=0  Ts=0
      settings: SourceProductBaseCode=PS
  Monostable3 : powerlib_meascontrol/Logic/Monostable  EdgeDetect=Rising  PulseDuration=3600  ic=0  Ts=0
      settings: SourceProductBaseCode=PS
  Mux : Mux  Inputs=2
  Rounding Function : Rounding  Operator=round
  Rounding Function1 : Rounding  Operator=round
  Unavailibilities : Outport
  tag scope: Unavailibilities=global
  wires:
  Add/1 -> Compare To Constant/1
  Monostable3/1 -> Data Type Conversion1/1
  Monostable2/1 -> Data Type Conversion2/1
  Data Type Conversion1/1 -> Gain4/1
  Compare To Constant/1 -> Logical Operator/1
  LessThanMin/1 -> Monostable3/1, Logical Operator1/1
  Logical Operator1/1 -> Logical Operator/2
  Data Type Conversion2/1 -> Gain2/1
  Integrator1/1 -> Rounding Function/1
  Integrator2/1 -> Rounding Function1/1
  Rounding Function/1 -> Mux/1
  Rounding Function1/1 -> Mux/2
  Mux/1 -> Unavailibilities/1, [Unavailibilities]
  Logical Operator/1 -> Monostable2/1
  Gain2/1 -> Integrator1/1
  Gain4/1 -> Integrator2/1
  Sat In/1 -> Add/1
  Sat Out/1 -> Add/2

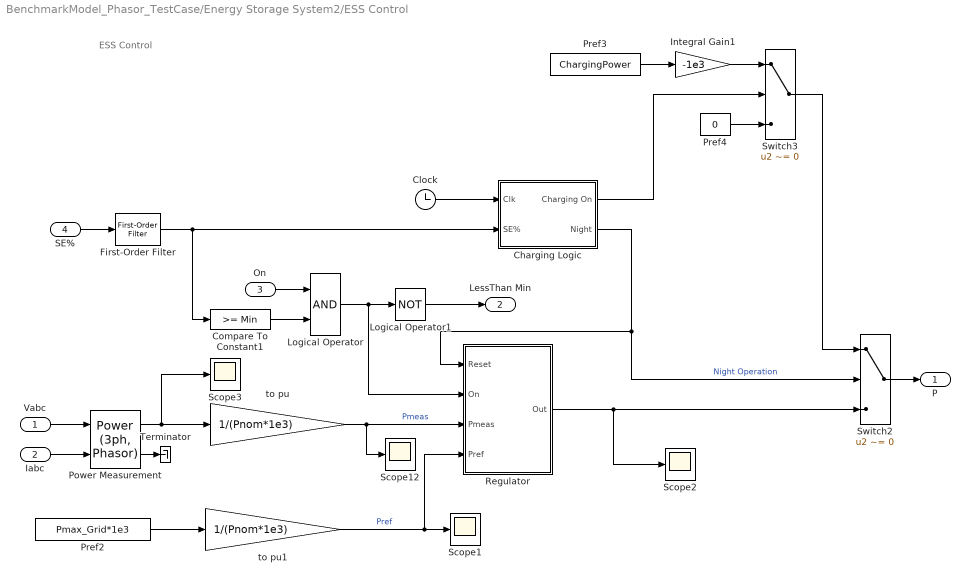
== system BenchmarkModel_Phasor_TestCase/Energy Storage System2/ESS Control ==
  note: ESS Control
  Vabc : Inport
  Iabc : Inport  Port=2
  On : Inport  Port=3
  SE% : Inport  Port=4
  Charging Logic : Subsystem
  Clock : Clock
  Compare To Constant1 : simulink/Logic and Bit Operations/Compare To Constant  relop=>=  const=Min  OutDataTypeStr=boolean
  First-Order Filter : powerlib_meascontrol/Filters/First-Order Filter  FilterType=Lowpass  Tc=1  Ts=0  Initialize=on  Vac_Init=[0, 0, 50]  Vdc_Init=Max  PlotResponse=off  FreqRange="[0,  200,  1]"
  Integral Gain1 : Gain  Gain=-1e3
  Logical Operator : Logic  AllPortsSameDT=off  OutDataTypeStr=boolean
  Logical Operator1 : Logic  Operator=NOT  AllPortsSameDT=off  OutDataTypeStr=boolean
  Power Measurement : powerlib_meascontrol/Measurements/Power (3ph, Phasor)
      settings: SourceProductBaseCode=PS
  Pref2 : Constant  Value=Pmax_Grid*1e3
  Pref3 : Constant  Value=ChargingPower
  Pref4 : Constant  Value=0
  Regulator : Subsystem
  Scope{1..3,12} (4 alike) : Scope
  Switch2 : Switch  Criteria=u2 ~= 0  Threshold=0.5
  Switch3 : Switch  Criteria=u2 ~= 0  Threshold=0.5
  Terminator : Terminator
  to pu : Gain  Gain=1/(Pnom*1e3)
  to pu1 : Gain  Gain=1/(Pnom*1e3)
  P : Outport  OutputWhenDisabled=reset  InitialOutput=0
  LessThan Min : Outport  Port=2  OutputWhenDisabled=reset  InitialOutput=0
  wires:
  Power Measurement/2 -> Terminator/1
  Vabc/1 -> Power Measurement/1
  Iabc/1 -> Power Measurement/2
  Power Measurement/1 -> Scope3/1, to pu/1
  Compare To Constant1/1 -> Logical Operator/2
  SE%/1 -> First-Order Filter/1
  Switch2/1 -> P/1
  Pref3/1 -> Integral Gain1/1
  On/1 -> Logical Operator/1
  Clock/1 -> Charging Logic/1(Clk)
  First-Order Filter/1 -> Compare To Constant1/1, Charging Logic/2(SE%)
  Logical Operator/1 -> Regulator/2(On), Logical Operator1/1
  Pref2/1 -> to pu1/1
  Logical Operator1/1 -> LessThan Min/1
  Integral Gain1/1 -> Switch3/1
  Pref4/1 -> Switch3/3
  Switch3/1 -> Switch2/1
  Charging Logic/2(Night) -> Regulator/1(Reset), Switch2/2  "Night Operation"
  Charging Logic/1(Charging On) -> Switch3/2
  to pu/1 -> Scope12/1, Regulator/3(Pmeas)  "Pmeas"
  to pu1/1 -> Regulator/4(Pref), Scope1/1  "Pref"
  Regulator/1(Out) -> Scope2/1, Switch2/3

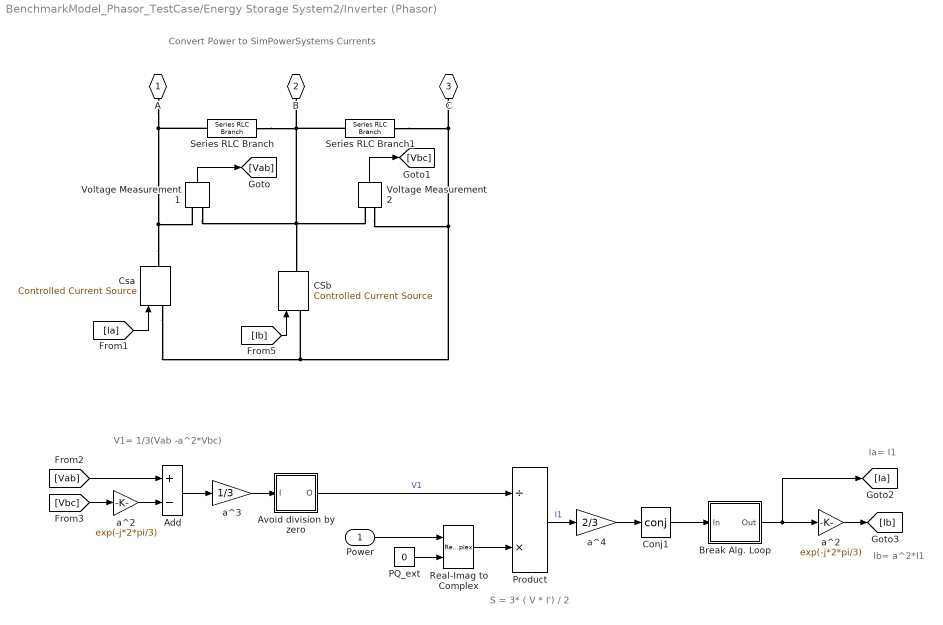
== system BenchmarkModel_Phasor_TestCase/Energy Storage System2/Inverter (Phasor) ==
  note: V1= 1/3(Vab -a^2*Vbc)
  note: S = 3* ( V * I') / 2
  note: Ia= I1
  note: Ib= a^2*I1
  note: Convert Power to SimPowerSystems Currents
  Power : Inport
  Add : Sum  Inputs=+-
  Avoid division by zero : Subsystem
  "Break Alg. Loop " : Subsystem
  CSb : powerlib/Electrical Sources/Controlled Current Source  Initialize=off  Source_Type=AC  Amplitude=0  Phase=0  Frequency=0  Measurements=None
  Conj1 : Math  Operator=conj  SignedPower=on  SaturateOnIntegerOverflow=on
  Csa : powerlib/Electrical Sources/Controlled Current Source  Initialize=off  Source_Type=AC  Amplitude=0  Phase=0  Frequency=0  Measurements=None
  PQ_ext : Constant  Value=0
  Product : Product  Inputs=/*  InputSameDT=on  SaturateOnIntegerOverflow=on  OutDataTypeStr=Inherit: Same as first input
  Real-Imag to Complex : RealImagToComplex
  Series RLC Branch : powerlib/Elements/Series RLC Branch  LConnTagsString=__new0  RConnTagsString=__new0  BranchType=R  Resistance=1e6  Inductance=1e-3  SetiL0=off  InitialCurrent=0  Capacitance=1e-6  Setx0=off  InitialVoltage=0  Measurements=None
  Series RLC Branch1 : powerlib/Elements/Series RLC Branch  LConnTagsString=__new0  RConnTagsString=__new0  BranchType=R  Resistance=1e6  Inductance=1e-3  SetiL0=off  InitialCurrent=0  Capacitance=1e-6  Setx0=off  InitialVoltage=0  Measurements=None
  Voltage Measurement1 : powerlib/Measurements/Voltage Measurement  PhasorSimulation=on  OutputType=Complex  PSBequivalent=0
  Voltage Measurement2 : powerlib/Measurements/Voltage Measurement  PhasorSimulation=on  OutputType=Complex  PSBequivalent=0
  a^2 : Gain  Gain=exp(-j*2*pi/3)  SaturateOnIntegerOverflow=on  OutDataTypeStr=Inherit: Same as input  ParamDataTypeStr=Inherit: Same as input
  "a^2 " : Gain  Gain=exp(-j*2*pi/3)  SaturateOnIntegerOverflow=on  OutDataTypeStr=Inherit: Same as input  ParamDataTypeStr=Inherit: Same as input
  a^3 : Gain  Gain=1/3  SaturateOnIntegerOverflow=on  OutDataTypeStr=Inherit: Same as input  ParamDataTypeStr=Inherit: Same as input
  a^4 : Gain  Gain=2/3  SaturateOnIntegerOverflow=on  OutDataTypeStr=Inherit: Same as input  ParamDataTypeStr=Inherit: Same as input
  A : PMIOPort  Tag=PMCPort  Side=Right
  B : PMIOPort  Tag=PMCPort  Port=2  Side=Right
  C : PMIOPort  Tag=PMCPort  Port=3  Side=Right
  wires:
  Power/1 -> Real-Imag to Complex/1
  Real-Imag to Complex/1 -> Product/2
  Product/1 -> a^4/1  "I1"
  PQ_ext/1 -> Real-Imag to Complex/2
  a^2/1 -> [Ib]
  Avoid division by zero/1(O) -> Product/1  "V1"
  Conj1/1 -> "Break Alg. Loop "/1(In)
  a^3/1 -> Avoid division by zero/1(I)
  Add/1 -> a^3/1
  [Vab] -> Add/1
  [Vbc] -> "a^2 "/1
  "a^2 "/1 -> Add/2
  a^4/1 -> Conj1/1
  "Break Alg. Loop "/1(Out) -> [Ia], a^2/1
  [Ib] -> CSb/1
  [Ia] -> Csa/1
  Voltage Measurement2/1 -> [Vbc]
  Voltage Measurement1/1 -> [Vab]
  connections:
  Series RLC Branch/RConn1 -- B/RConn1 -- Series RLC Branch1/LConn1 -- CSb/RConn1 -- Voltage Measurement1/LConn2 -- Voltage Measurement2/LConn1
  Series RLC Branch1/RConn1 -- C/RConn1 -- Csa/LConn1 -- CSb/LConn1 -- Voltage Measurement2/LConn2
  Csa/RConn1 -- A/RConn1 -- Series RLC Branch/LConn1 -- Voltage Measurement1/LConn1

== system BenchmarkModel_Phasor_TestCase/Energy Storage System2/Stored Energy Calculation (%) ==
  Pin : Inport
  Charge : Gain  Gain=Efficiency/100
  Compare To Zero : simulink/Logic and Bit Operations/Compare To Zero  relop=<=  OutDataTypeStr=boolean
  Constant : Constant  Value=kWh_Rated
  Discharge : Gain  Gain=1/(Efficiency/100)
  Divide : Product  Inputs=*/
  Gain3 : Gain  Gain=1/3600/1e3
  Gain5 : Gain  Gain=-1
  Integrator : Integrator  InitialCondition=(Initial_kWh_pc/100)*kWh_Rated*3600*1e3
  Switch1 : Switch  Criteria=u2 ~= 0
  Transfer Fcn : TransferFcn  Denominator=[1 1]
  to % : Gain  Gain=100
  SE% : Outport
  wires:
  Pin/1 -> Charge/1, Discharge/1, Transfer Fcn/1
  Integrator/1 -> Gain3/1
  Compare To Zero/1 -> Switch1/2
  Divide/1 -> to %/1
  Charge/1 -> Switch1/1
  Constant/1 -> Divide/2
  Gain3/1 -> Divide/1
  Switch1/1 -> Gain5/1
  Transfer Fcn/1 -> Compare To Zero/1
  to %/1 -> SE%/1
  Gain5/1 -> Integrator/1
  Discharge/1 -> Switch1/3

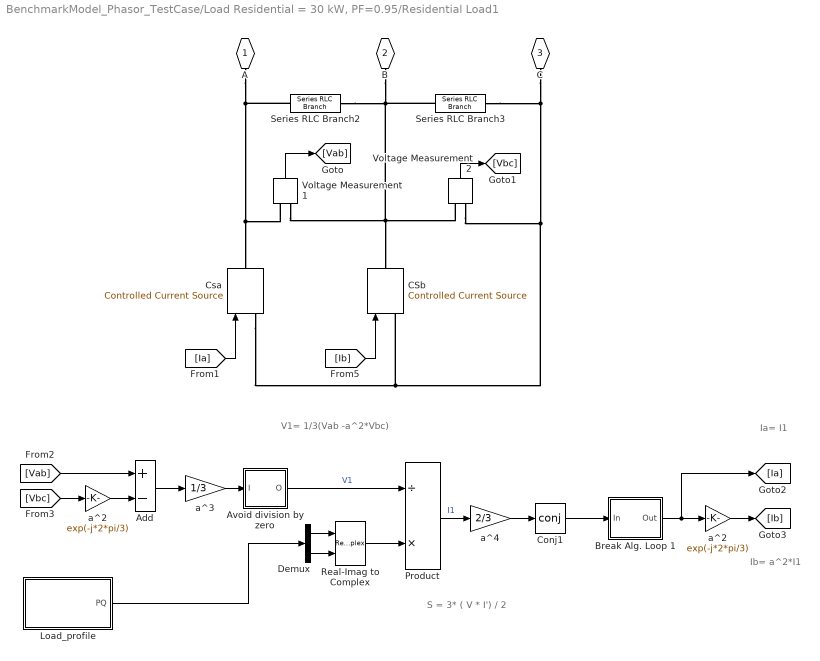
== system BenchmarkModel_Phasor_TestCase/Load Residential = 30 kW, PF=0.95/Residential Load1 ==
  note: Ib= a^2*I1
  note: Ia= I1
  note: S = 3* ( V * I') / 2
  note: V1= 1/3(Vab -a^2*Vbc)
  Add : Sum  Inputs=+-
  Avoid division by zero : Subsystem
  Break Alg. Loop 1 : Subsystem
  CSb : powerlib/Electrical Sources/Controlled Current Source  Initialize=on  Source_Type=AC  Amplitude=10  Phase=(2.751-2*pi/3)*180/pi  Frequency=50  Measurements=Current
  Conj1 : Math  Operator=conj  SignedPower=on  SaturateOnIntegerOverflow=on
  Csa : powerlib/Electrical Sources/Controlled Current Source  Initialize=on  Source_Type=AC  Amplitude=10  Phase=2.751*180/pi  Frequency=50  Measurements=Current
  Demux : Demux  Outputs=2
  Load_profile : Subsystem
  Product : Product  Inputs=/*  InputSameDT=on  SaturateOnIntegerOverflow=on  OutDataTypeStr=Inherit: Same as first input
  Real-Imag to Complex : RealImagToComplex
  Series RLC Branch2 : powerlib/Elements/Series RLC Branch  LConnTagsString=__new0  RConnTagsString=__new0  BranchType=R  Resistance=1e6  Inductance=1e-3  SetiL0=off  InitialCurrent=0  Capacitance=1e-6  Setx0=off  InitialVoltage=0  Measurements=None
  Series RLC Branch3 : powerlib/Elements/Series RLC Branch  LConnTagsString=__new0  RConnTagsString=__new0  BranchType=R  Resistance=1e6  Inductance=1e-3  SetiL0=off  InitialCurrent=0  Capacitance=1e-6  Setx0=off  InitialVoltage=0  Measurements=None
  Voltage Measurement1 : powerlib/Measurements/Voltage Measurement  PhasorSimulation=on  OutputType=Complex  PSBequivalent=0
  Voltage Measurement2 : powerlib/Measurements/Voltage Measurement  PhasorSimulation=on  OutputType=Complex  PSBequivalent=0
  a^2 : Gain  Gain=exp(-j*2*pi/3)  SaturateOnIntegerOverflow=on  OutDataTypeStr=Inherit: Same as input  ParamDataTypeStr=Inherit: Same as input
  "a^2 " : Gain  Gain=exp(-j*2*pi/3)  SaturateOnIntegerOverflow=on  OutDataTypeStr=Inherit: Same as input  ParamDataTypeStr=Inherit: Same as input
  a^3 : Gain  Gain=1/3  SaturateOnIntegerOverflow=on  OutDataTypeStr=Inherit: Same as input  ParamDataTypeStr=Inherit: Same as input
  a^4 : Gain  Gain=2/3  SaturateOnIntegerOverflow=on  OutDataTypeStr=Inherit: Same as input  ParamDataTypeStr=Inherit: Same as input
  A : PMIOPort  Tag=PMCPort  Side=Left
  B : PMIOPort  Tag=PMCPort  Port=2  Side=Left
  C : PMIOPort  Tag=PMCPort  Port=3  Side=Left
  wires:
  Break Alg. Loop 1/1(Out) -> [Ia], a^2/1
  [Ib] -> CSb/1
  Conj1/1 -> Break Alg. Loop 1/1(In)
  a^2/1 -> [Ib]
  Avoid division by zero/1(O) -> Product/1  "V1"
  Add/1 -> a^3/1
  Voltage Measurement2/1 -> [Vbc]
  Product/1 -> a^4/1  "I1"
  Voltage Measurement1/1 -> [Vab]
  [Vbc] -> "a^2 "/1
  [Ia] -> Csa/1
  a^4/1 -> Conj1/1
  [Vab] -> Add/1
  Demux/1 -> Real-Imag to Complex/1
  "a^2 "/1 -> Add/2
  Real-Imag to Complex/1 -> Product/2
  Demux/2 -> Real-Imag to Complex/2
  a^3/1 -> Avoid division by zero/1(I)
  Load_profile/1(PQ) -> Demux/1
  connections:
  Series RLC Branch2/RConn1 -- CSb/RConn1 -- Voltage Measurement2/LConn1 -- Voltage Measurement1/LConn2 -- B/RConn1 -- Series RLC Branch3/LConn1
  Series RLC Branch3/RConn1 -- Voltage Measurement2/LConn2 -- Csa/LConn1 -- CSb/LConn1 -- C/RConn1
  Voltage Measurement1/LConn1 -- Csa/RConn1 -- Series RLC Branch2/LConn1 -- A/RConn1

== system BenchmarkModel_Phasor_TestCase/OLTC/Seq.An ==
  abc : Inport
  Sequence Analyzer (Phasor) : powerlib_meascontrol/Measurements/Sequence Analyzer (Phasor)  seq=Positive
      settings: SourceProductBaseCode=PS
  Terminator : Terminator
  Mag : Outport
  wires:
  abc/1 -> Sequence Analyzer (Phasor)/1
  Sequence Analyzer (Phasor)/2 -> Terminator/1
  Sequence Analyzer (Phasor)/1 -> Mag/1

== system BenchmarkModel_Phasor_TestCase/OLTC/Seq.An2 ==
  abc : Inport
  Sequence Analyzer (Phasor) : powerlib_meascontrol/Measurements/Sequence Analyzer (Phasor)  seq=Positive
      settings: SourceProductBaseCode=PS
  Terminator : Terminator
  Mag : Outport
  wires:
  abc/1 -> Sequence Analyzer (Phasor)/1
  Sequence Analyzer (Phasor)/2 -> Terminator/1
  Sequence Analyzer (Phasor)/1 -> Mag/1

== system BenchmarkModel_Phasor_TestCase/OLTC/Seq.An3 ==
  abc : Inport
  Sequence Analyzer (Phasor) : powerlib_meascontrol/Measurements/Sequence Analyzer (Phasor)  seq=Positive
      settings: SourceProductBaseCode=PS
  Terminator : Terminator
  Mag : Outport
  wires:
  abc/1 -> Sequence Analyzer (Phasor)/1
  Sequence Analyzer (Phasor)/2 -> Terminator/1
  Sequence Analyzer (Phasor)/1 -> Mag/1
